simulink model "SimulacaoPID"  (R2020a)
settings: Solver=VariableStepAuto  StartTime=0.0  StopTime=80  RelTol=1e-3
values from neighbouring files (symbols this model uses):
  b = [1 0 0]    [Exemple_3_disertacao.mat]    (also in Exemple_4_disertacao.mat = [1 0])
  C = [1  -0.9999; -0.9999  1]    [Exemple_3_disertacao.mat]    (also in Exemple_4_disertacao.mat = [1  -0.9; -1  1])
  K = [1500  -500  0; -500  600  -100; 0  -100  100]    [Exemple_3_disertacao.mat]    (also in Exemple_4_disertacao.mat = [3  -2; -2  3])
  kd = 1.58696632955    [Exemple_3_disertacao.mat]    (also in Exemple_4_disertacao.mat = 0.73545354663; plots.m = melhor_individuo(3); run.m = melhor_individuo(3))
  ki = 0.157850360777    [Exemple_3_disertacao.mat]    (also in Exemple_4_disertacao.mat = 2.32478302823; plots.m = melhor_individuo(2); run.m = melhor_individuo(2))
  kp = 1.19418417659    [Exemple_3_disertacao.mat]    (also in Exemple_4_disertacao.mat = 2.62011638281; plots.m = melhor_individuo(1); run.m = melhor_individuo(1))
  M = [10  0  0; 0  10  0; 0  0  10]    [Exemple_3_disertacao.mat]    (also in Exemple_4_disertacao.mat = [1  0; 0  1])
  tau = 0.7    [Exemple_3_disertacao.mat]    (also in Exemple_4_disertacao.mat = 0.5)
undefined symbols (not defined in the file or in its folder): l
settings Model: Creator=Dantas  LastModifiedBy=jhona
settings DataIOCC: ReturnWorkspaceOutputs=off
settings DebuggingCC: ArithmeticOperatorsInVariantConditions=warning
settings SFSimCC: SimUseLocalCustomCode=off  CustomCodeUndefinedFunction=UseInterfaceOnly
settings RTWCC: RTWUseLocalCustomCode=off
settings CodeAppCC: StateflowObjectComments=on

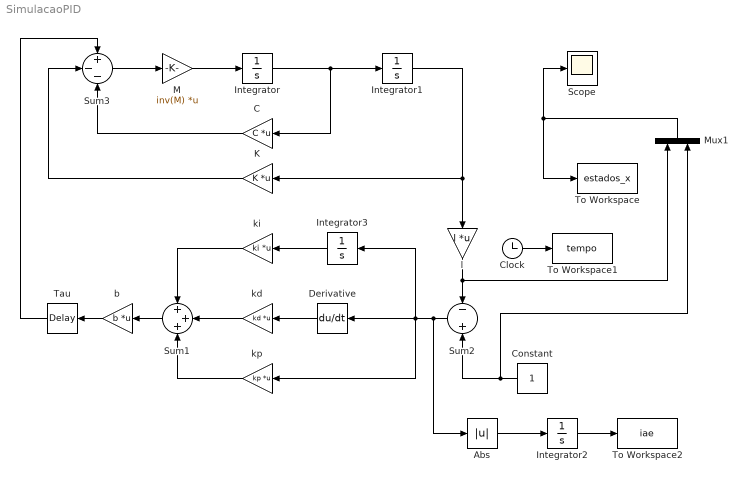
== system SimulacaoPID ==
  Abs : Abs
  C : Gain  Gain=C  Multiplication=Matrix(K*u)
  Clock : Clock
  Constant : Constant
  Derivative : Derivative
  Integrator{,1..3} (4 alike) : Integrator
  K : Gain  Gain=K  Multiplication=Matrix(K*u)
  M : Gain  Gain=inv(M)  Multiplication=Matrix(K*u)
  Mux1 : Mux  Inputs=2
  Scope : Scope
  Sum1 : Sum  Inputs=+++
  Sum2 : Sum  Inputs=-|+
  Sum3 : Sum  Inputs=+--
  Tau : TransportDelay  DelayTime=tau
  To Workspace : ToWorkspace  VariableName=estados_x  SampleTime=-1
  To Workspace1 : ToWorkspace  VariableName=tempo  SampleTime=-1
  To Workspace2 : ToWorkspace  VariableName=iae  SampleTime=-1
  b : Gain  Gain=b  Multiplication=Matrix(K*u)
  kd : Gain  Gain=kd  Multiplication=Matrix(K*u)
  ki : Gain  Gain=ki  Multiplication=Matrix(K*u)
  kp : Gain  Gain=kp  Multiplication=Matrix(K*u)
  l : Gain  Gain=l  Multiplication=Matrix(K*u)
  wires:
  Sum3/1 -> M/1
  M/1 -> Integrator/1
  Integrator1/1 -> l/1, K/1
  Integrator/1 -> C/1, Integrator1/1
  C/1 -> Sum3/3
  K/1 -> Sum3/2
  Clock/1 -> To Workspace1/1
  Integrator3/1 -> ki/1
  ki/1 -> Sum1/1
  kd/1 -> Sum1/2
  kp/1 -> Sum1/3
  Sum1/1 -> b/1
  b/1 -> Tau/1
  Tau/1 -> Sum3/1
  Constant/1 -> Mux1/2, Sum2/2
  Sum2/1 -> Abs/1, Integrator3/1, kp/1, Derivative/1
  Derivative/1 -> kd/1
  l/1 -> Mux1/1, Sum2/1
  Abs/1 -> Integrator2/1
  Integrator2/1 -> To Workspace2/1
  Mux1/1 -> To Workspace/1, Scope/1
